simulink model "Kalman_testenv"  (R2019a)
settings: Solver=FixedStepAuto  StartTime=0.0  StopTime=30  FixedStep=Ts  RelTol=1e-3
values from neighbouring files (symbols this model uses):
  measnoiseamp = 0.01    [Kalman_testenv_i.m]
  Ts = 1e-3    (= 0.001)    [Kalman_testenv_i.m]
undefined symbols (not defined in the file or in its folder): DiscIntNeverNeededParam, Discrete, msd, Time, vdp, xhat0
libraries: simulink x2, sharedTrackingLibrary x1, ctrlSharedLib x1
settings Model: Creator=Daniel  LastModifiedBy=Daniel

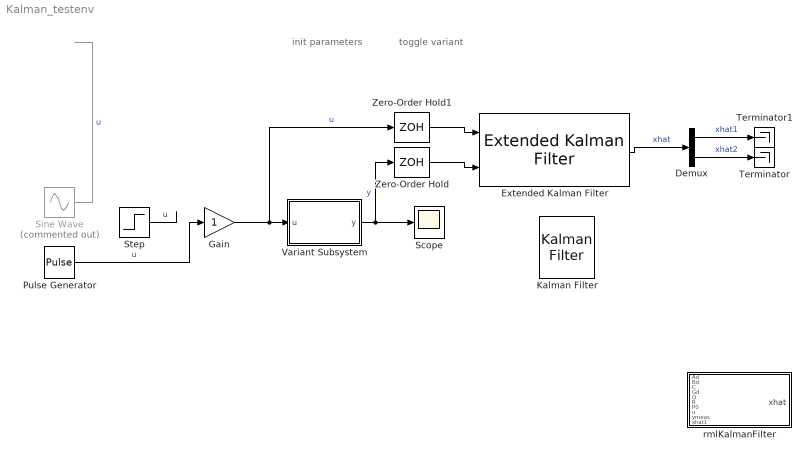
== system Kalman_testenv ==
  note: init parameters
  note: toggle variant
  Demux : Demux  Outputs=2
  Extended Kalman Filter : sharedTrackingLibrary/Extended Kalman Filter  StateTransitionFcn=Msd_Kalman_state  HasStateTransitionJacobianFcn=off  HasAdditiveProcessNoise=Additive  ProcessNoise=1  HasTimeVaryingProcessNoise=off  HasStateTransitionFcnExtraArgument=1  InitialState=[5;0]  InitialStateCovariance=1  MeasurementFcn1=Msd_Kalman_out  HasMeasurementJacobianFcn1=off  HasMeasurementEnablePort1=off  HasAdditiveMeasurementNoise1=Additive  MeasurementNoise1=0.1  HasTimeVaryingMeasurementNoise1=off  HasMeasurementFcnExtraArgument1=0  MeasurementFcn2=myMeasurementFcn  HasMeasurementJacobianFcn2=off  HasMeasurementEnablePort2=off  HasAdditiveMeasurementNoise2=Additive  MeasurementNoise2=1  HasTimeVaryingMeasurementNoise2=off  HasMeasurementFcnExtraArgument2=0  MeasurementFcn3=myMeasurementFcn  HasMeasurementJacobianFcn3=off  HasMeasurementEnablePort3=off  HasAdditiveMeasurementNoise3=Additive  MeasurementNoise3=1  HasTimeVaryingMeasurementNoise3=off  HasMeasurementFcnExtraArgument3=0  MeasurementFcn4=myMeasurementFcn  HasMeasurementJacobianFcn4=off  HasMeasurementEnablePort4=off  HasAdditiveMeasurementNoise4=Additive  MeasurementNoise4=1  HasTimeVaryingMeasurementNoise4=off  HasMeasurementFcnExtraArgument4=0  MeasurementFcn5=myMeasurementFcn  HasMeasurementJacobianFcn5=off  HasMeasurementEnablePort5=off  HasAdditiveMeasurementNoise5=Additive  MeasurementNoise5=1  HasTimeVaryingMeasurementNoise5=off  HasMeasurementFcnExtraArgument5=0  EnableMultirate=off  StateTransitionFcnSampleTime=1  MeasurementFcn1SampleTime=1  MeasurementFcn2SampleTime=1  MeasurementFcn3SampleTime=1  MeasurementFcn4SampleTime=1  MeasurementFcn5SampleTime=1  UseCurrentEstimator=on  OutputStateCovariance=off  DataType=double  SampleTime=Ts  NumberOfMeasurements=1
      settings: SourceProductName=Control System Toolbox  SourceProductBaseCode=CT
  Gain : Gain
  Kalman Filter : ctrlSharedLib/Kalman Filter  TimeDomain=Discrete-Time  UseCurrentEstimator=on  ModelSource=LTI State-Space Variable  ModelSourceVariable=ss(0.95,1,1,0,1)  A=0.95  B=1  C=1  D=0  NumberOfStates=1  NumberOfInputs=1  NumberOfOutputs=1  InitialEstimateSource=Dialog  X0=0  P0=10  UseK=off  UseGH=off  NumberOfProcessNoiseInputs=1  G=1  TimeInvariantG=on  H=0  TimeInvariantH=on  Q=0.05  TimeInvariantQ=on  R=1  TimeInvariantR=on  N=0  TimeInvariantN=on  AddInputPort=on  AddEnablePort=off  OutputEstimatedY=off  OutputP=off  Ts=-1
      settings: SourceProductBaseCode=CT
  Pulse Generator : DiscretePulseGenerator  PulseType=Time based  Amplitude=0  Period=100
  Scope : Scope
  Sine Wave : Sin  Commented=on  Amplitude=1e-3  Frequency=1.15  SampleTime=0
  Step : Step  Time=3  After=5  SampleTime=0
  Terminator : Terminator
  Terminator1 : Terminator
  Variant Subsystem : Subsystem  Variant=on
  Zero-Order Hold : ZeroOrderHold  SampleTime=Ts
  Zero-Order Hold1 : ZeroOrderHold  SampleTime=Ts
  rmlKalmanFilter : Subsystem
  wires:
  Gain/1 -> Variant Subsystem/1(u), Zero-Order Hold1/1  "u"
  Variant Subsystem/1(y) -> Scope/1, Zero-Order Hold/1  "y"
  Extended Kalman Filter/1 -> Demux/1  "xhat"
  Zero-Order Hold/1 -> Extended Kalman Filter/2
  Zero-Order Hold1/1 -> Extended Kalman Filter/1
  Demux/1 -> Terminator1/1  "xhat1"
  Demux/2 -> Terminator/1  "xhat2"
  Sine Wave/1 -> ?  "u"
  Step/1 -> ?  "u"
  Pulse Generator/1 -> Gain/1  "u"

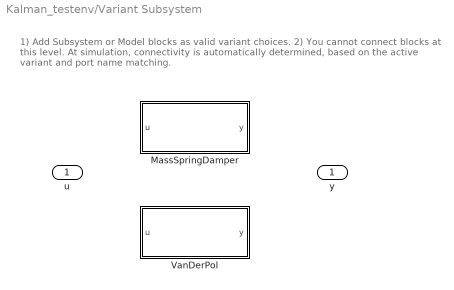
== system Kalman_testenv/Variant Subsystem ==
  note: 1) Add Subsystem or Model blocks as valid variant choices.
      | 2) You cannot connect blocks at this level. At simulation, connectivity is automatically
      | determined, based on the active variant and port name matching.
  u : Inport
  MassSpringDamper : Subsystem  VariantControl=thisMode == 0
  VanDerPol : Subsystem  VariantControl=thisMode == 1
  y : Outport

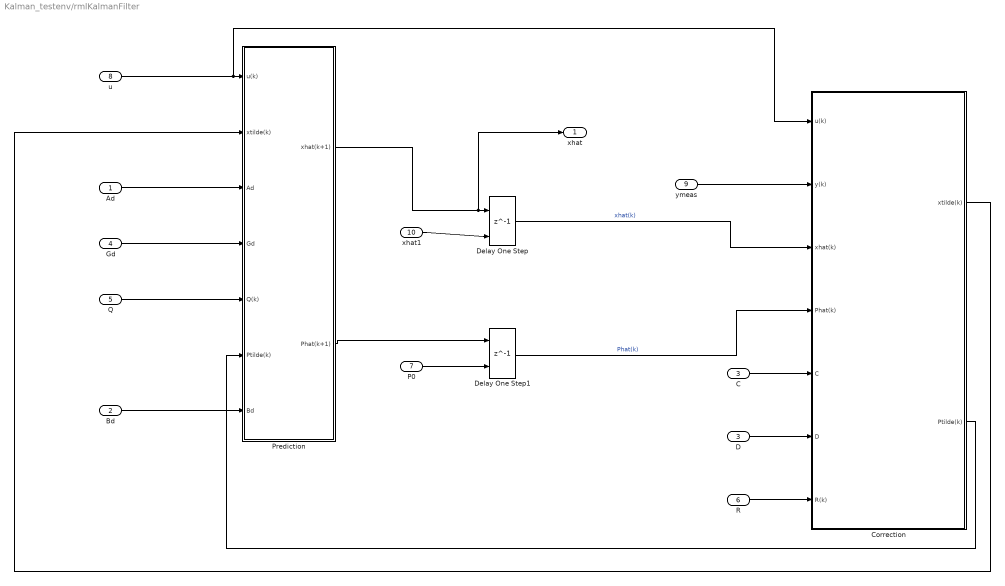
== system Kalman_testenv/rmlKalmanFilter ==
  Ad : Inport
  Bd : Inport  Port=2
  C : Inport  Port=3
  Gd : Inport  Port=4
  Q : Inport  Port=5
  R : Inport  Port=6
  P0 : Inport  Port=7
  u : Inport  Port=8
  ymeas : Inport  Port=9
  xhat1 : Inport  Port=10
  Correction : Subsystem
  D : InportShadow  Port=3
  Delay One Step : Delay  DelayLength=1  InitialConditionSource=Input port  InitialCondition=xhat0
      settings: InputPortMap=u0,p4
  Delay One Step1 : Delay  DelayLength=1  InitialConditionSource=Input port  InitialCondition=xhat0
      settings: InputPortMap=u0,p4
  Prediction : Subsystem
  xhat : Outport
  wires:
  Delay One Step/1 -> Correction/3(xhat(k))  "xhat(k)"
  P0/1 -> Delay One Step1/2
  Delay One Step1/1 -> Correction/4(Phat(k))  "Phat(k)"
  u/1 -> Correction/1(u(k)), Prediction/1(u(k))
  Correction/1(xtilde(k)) -> Prediction/2(xtilde(k))
  Ad/1 -> Prediction/3(Ad)
  Gd/1 -> Prediction/4(Gd)
  Q/1 -> Prediction/5(Q(k))
  Correction/2(Ptilde(k)) -> Prediction/6(Ptilde(k))
  Prediction/1(xhat(k+1)) -> xhat/1, Delay One Step/1
  xhat1/1 -> Delay One Step/2
  Prediction/2(Phat(k+1)) -> Delay One Step1/1
  ymeas/1 -> Correction/2(y(k))
  C/1 -> Correction/5(C)
  Bd/1 -> Prediction/7(Bd)
  D/1 -> Correction/6(D)
  R/1 -> Correction/7(R(k))

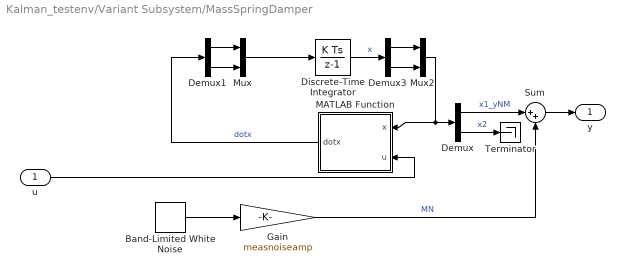
== system Kalman_testenv/Variant Subsystem/MassSpringDamper ==
  u : Inport
  Band-Limited White Noise : simulink/Sources/Band-Limited White Noise  Cov=1  Ts=0.01  seed=[23341]
  Demux : Demux  Outputs=2
  Demux1 : Demux  Outputs=2
  Demux3 : Demux  Outputs=2
  Discrete-Time Integrator : DiscreteIntegrator  InitialCondition=[msd.x0, 0]  SampleTime=-1  ICPrevOutput=DiscIntNeverNeededParam  ICPrevScaledInput=DiscIntNeverNeededParam
  Gain : Gain  Gain=measnoiseamp
  MATLAB Function : MATLAB Function  TreatAsAtomicUnit=on
  Mux : Mux  Inputs=2
  Mux2 : Mux  Inputs=2
  Sum : Sum  Inputs=|++
  Terminator : Terminator
  y : Outport
  wires:
  u/1 -> MATLAB Function/2(u)
  Sum/1 -> y/1
  Demux3/2 -> Mux2/2
  Demux3/1 -> Mux2/1
  MATLAB Function/1(dotx) -> Demux1/1  "dotx"
  Discrete-Time Integrator/1 -> Demux3/1  "x"
  Gain/1 -> Sum/2  "MN"
  Demux/2 -> Terminator/1  "x2"
  Demux/1 -> Sum/1  "x1_yNM"
  Demux1/2 -> Mux/2
  Mux2/1 -> Demux/1, MATLAB Function/1(x)
  Band-Limited White Noise/1 -> Gain/1
  Mux/1 -> Discrete-Time Integrator/1
  Demux1/1 -> Mux/1

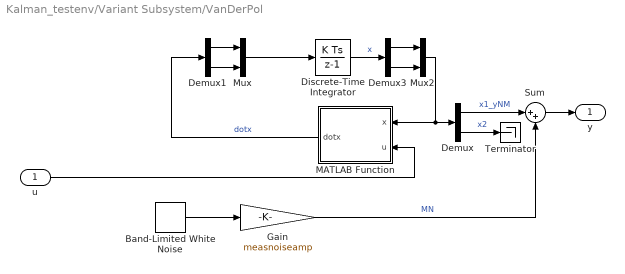
== system Kalman_testenv/Variant Subsystem/VanDerPol ==
  u : Inport
  Band-Limited White Noise : simulink/Sources/Band-Limited White Noise  Cov=1  Ts=0.01  seed=[23341]
  Demux : Demux  Outputs=2
  Demux1 : Demux  Outputs=2
  Demux3 : Demux  Outputs=2
  Discrete-Time Integrator : DiscreteIntegrator  InitialCondition=[vdp.x0;0]  SampleTime=-1  ICPrevOutput=DiscIntNeverNeededParam  ICPrevScaledInput=DiscIntNeverNeededParam
  Gain : Gain  Gain=measnoiseamp
  MATLAB Function : MATLAB Function  TreatAsAtomicUnit=on
  Mux : Mux  Inputs=2
  Mux2 : Mux  Inputs=2
  Sum : Sum  Inputs=|++
  Terminator : Terminator
  y : Outport
  wires:
  Demux1/1 -> Mux/1
  Mux2/1 -> Demux/1, MATLAB Function/1(x)
  Gain/1 -> Sum/2  "MN"
  Demux1/2 -> Mux/2
  Band-Limited White Noise/1 -> Gain/1
  Mux/1 -> Discrete-Time Integrator/1
  Demux/2 -> Terminator/1  "x2"
  Sum/1 -> y/1
  Demux/1 -> Sum/1  "x1_yNM"
  Demux3/1 -> Mux2/1
  u/1 -> MATLAB Function/2(u)
  Demux3/2 -> Mux2/2
  Discrete-Time Integrator/1 -> Demux3/1  "x"
  MATLAB Function/1(dotx) -> Demux1/1  "dotx"

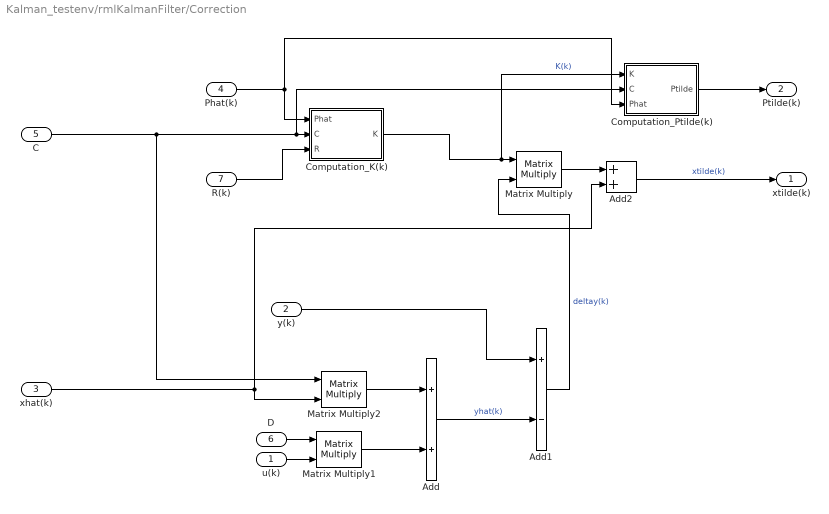
== system Kalman_testenv/rmlKalmanFilter/Correction ==
  u(k) : Inport
  y(k) : Inport  Port=2
  xhat(k) : Inport  Port=3
  Phat(k) : Inport  Port=4
  C : Inport  Port=5
  D : Inport  Port=6
  R(k) : Inport  Port=7
  Add : Sum
  Add1 : Sum  Inputs=+-
  Add2 : Sum
  Computation_K(k) : MATLAB Function  TreatAsAtomicUnit=on
  Computation_Ptilde(k) : MATLAB Function  TreatAsAtomicUnit=on
  Matrix Multiply : Product  Multiplication=Matrix(*)
  Matrix Multiply1 : Product  Multiplication=Matrix(*)
  Matrix Multiply2 : Product  Multiplication=Matrix(*)
  xtilde(k) : Outport
  Ptilde(k) : Outport  Port=2
  wires:
  Add/1 -> Add1/2  "yhat(k)"
  xhat(k)/1 -> Add2/2, Matrix Multiply2/2
  Matrix Multiply2/1 -> Add/1
  u(k)/1 -> Matrix Multiply1/2
  y(k)/1 -> Add1/1
  Add1/1 -> Matrix Multiply/2  "deltay(k)"
  Computation_K(k)/1(K) -> Computation_Ptilde(k)/1(K), Matrix Multiply/1  "K(k)"
  Phat(k)/1 -> Computation_K(k)/1(Phat), Computation_Ptilde(k)/3(Phat)
  C/1 -> Computation_Ptilde(k)/2(C), Computation_K(k)/2(C), Matrix Multiply2/1
  R(k)/1 -> Computation_K(k)/3(R)
  Matrix Multiply/1 -> Add2/1
  Add2/1 -> xtilde(k)/1  "xtilde(k)"
  Computation_Ptilde(k)/1(Ptilde) -> Ptilde(k)/1
  D/1 -> Matrix Multiply1/1
  Matrix Multiply1/1 -> Add/2

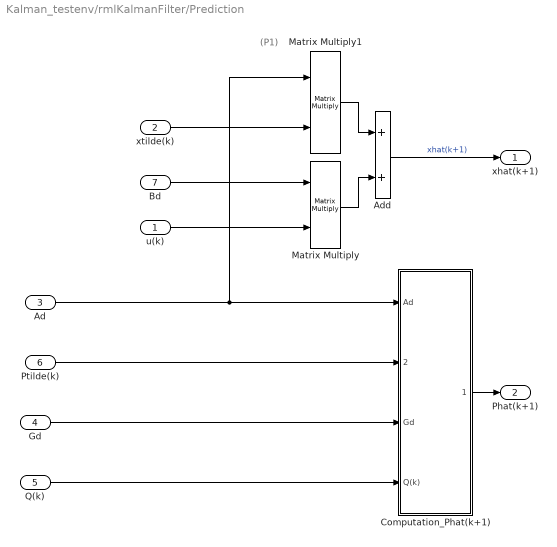
== system Kalman_testenv/rmlKalmanFilter/Prediction ==
  note: (P1)
  u(k) : Inport
  xtilde(k) : Inport  Port=2
  Ad : Inport  Port=3
  Gd : Inport  Port=4
  Q(k) : Inport  Port=5
  Ptilde(k) : Inport  Port=6
  Bd : Inport  Port=7
  Add : Sum
  Computation_Phat(k+1) : Subsystem
  Matrix Multiply : Product  Multiplication=Matrix(*)
  Matrix Multiply1 : Product  Multiplication=Matrix(*)
  xhat(k+1) : Outport
  Phat(k+1) : Outport  Port=2
  wires:
  Computation_Phat(k+1)/1(Phat(k+1)) -> Phat(k+1)/1
  Matrix Multiply1/1 -> Add/1
  Ptilde(k)/1 -> Computation_Phat(k+1)/2(Ptilde(k))
  Matrix Multiply/1 -> Add/2
  u(k)/1 -> Matrix Multiply/2
  Gd/1 -> Computation_Phat(k+1)/3(Gd)
  Add/1 -> xhat(k+1)/1  "xhat(k+1)"
  Ad/1 -> Computation_Phat(k+1)/1(Ad), Matrix Multiply1/1
  Q(k)/1 -> Computation_Phat(k+1)/4(Q(k))
  xtilde(k)/1 -> Matrix Multiply1/2
  Bd/1 -> Matrix Multiply/1

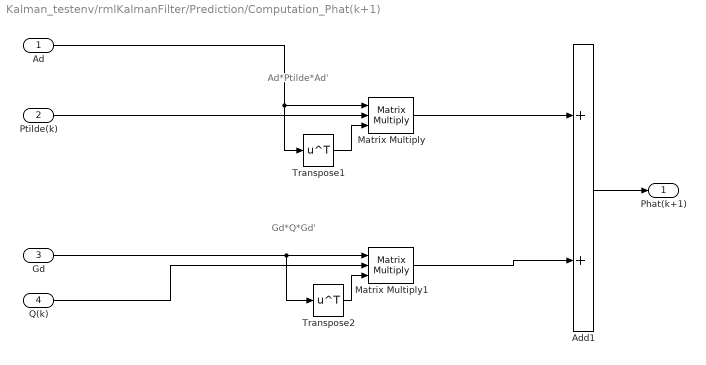
== system Kalman_testenv/rmlKalmanFilter/Prediction/Computation_Phat(k+1) ==
  note: Gd*Q*Gd'
  note: Ad*Ptilde*Ad'
  Ad : Inport
  Ptilde(k) : Inport  Port=2
  Gd : Inport  Port=3
  Q(k) : Inport  Port=4
  Add1 : Sum
  Matrix Multiply : Product  Inputs=3  Multiplication=Matrix(*)
  Matrix Multiply1 : Product  Inputs=3  Multiplication=Matrix(*)
  Transpose1 : Math  Operator=transpose  SaturateOnIntegerOverflow=on
  Transpose2 : Math  Operator=transpose  SaturateOnIntegerOverflow=on
  Phat(k+1) : Outport
  wires:
  Transpose1/1 -> Matrix Multiply/3
  Matrix Multiply/1 -> Add1/1
  Add1/1 -> Phat(k+1)/1
  Matrix Multiply1/1 -> Add1/2
  Transpose2/1 -> Matrix Multiply1/3
  Gd/1 -> Transpose2/1, Matrix Multiply1/1
  Ptilde(k)/1 -> Matrix Multiply/2
  Ad/1 -> Transpose1/1, Matrix Multiply/1
  Q(k)/1 -> Matrix Multiply1/2

== matlab function Kalman_testenv/Variant Subsystem/VanDerPol/MATLAB Function ==
  data: x input; u input; dotx output; vdp parameter
function dotx = fcn(x,u,vdp)
   mue = vdp.mue;
    dotx = zeros(2,1);
    dotx = [x(2); mue.*(1-x(1)^2)*x(2)-x(1) + u];
end

== matlab function Kalman_testenv/Variant Subsystem/MassSpringDamper/MATLAB Function ==
  data: x input; u input; dotx output; msd parameter
function dotx = fcn(x,u,msd)
k = msd.k; m = msd.m; d = msd.d;
    dotx = zeros(2,1);
    dotx =[ x(2); -d/m*x(2)-k/m*x(1)-1/m*u];
end

== matlab function Kalman_testenv/rmlKalmanFilter/Correction/Computation_K(k) ==
  data: Phat input; K output; C input; R input
function K = fcn(Phat, C, R)
   K = Phat*C'*inv(C*Phat*C' + R);
end

== matlab function Kalman_testenv/rmlKalmanFilter/Correction/Computation_Ptilde(k) ==
  data: K input; Ptilde output; C input; Phat input
function Ptilde = fcn(K,C,Phat)
    I = eye(size(K,1));
    Ptilde = (I- K*C)*Phat;
end
